simulink model "teste2"  (R2014a)
settings: Solver=ode3  StartTime=0.0  StopTime=80  FixedStep=0.001  RelTol=1e-3
libraries: commchan3 x3, simulink x2
settings Model: Creator=andre  LastModifiedBy=andre

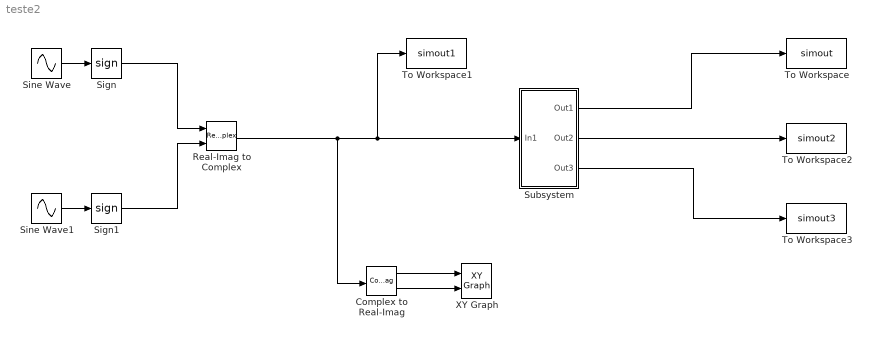
== system teste2 ==
  Complex to Real-Imag : ComplexToRealImag
  Real-Imag to Complex : RealImagToComplex
  Sign : Signum
  Sign1 : Signum
  Sine Wave : Sin  Frequency=10  Phase=0.15  SampleTime=0
  Sine Wave1 : Sin  Frequency=3  Phase=-0.17  SampleTime=0
  Subsystem : Subsystem
  To Workspace : ToWorkspace  VariableName=simout  SampleTime=-1
  To Workspace1 : ToWorkspace  VariableName=simout1  SampleTime=-1
  To Workspace2 : ToWorkspace  VariableName=simout2  SampleTime=-1
  To Workspace3 : ToWorkspace  VariableName=simout3  SampleTime=-1
  XY Graph : simulink/Sinks/XY Graph  xmin=-3  xmax=3  ymin=-3  ymax=3  st=-1
  wires:
  Sine Wave/1 -> Sign/1
  Sine Wave1/1 -> Sign1/1
  Subsystem/1(Out1) -> To Workspace/1
  Subsystem/2(Out2) -> To Workspace2/1
  Subsystem/3(Out3) -> To Workspace3/1
  Sign/1 -> Real-Imag to Complex/1
  Sign1/1 -> Real-Imag to Complex/2
  Complex to Real-Imag/1 -> XY Graph/1
  Complex to Real-Imag/2 -> XY Graph/2
  Real-Imag to Complex/1 -> Complex to Real-Imag/1, To Workspace1/1, Subsystem/1(In1)

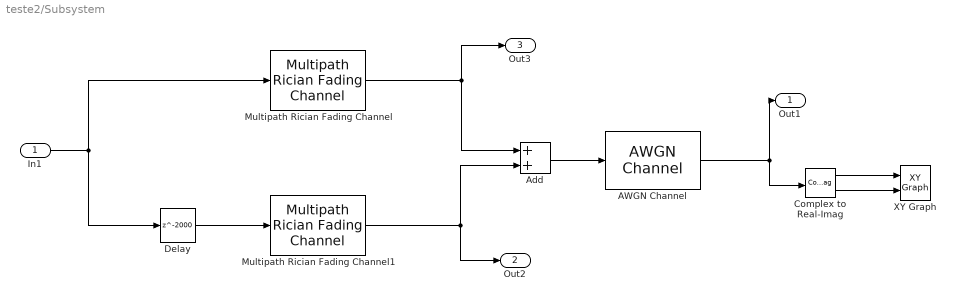
== system teste2/Subsystem ==
  In1 : Inport
  AWGN Channel : commchan3/AWGN Channel  InputProcessing=Inherited (this choice will be removed - see release notes)  seed=67  noiseMode="Signal to noise ratio  (SNR)"  EbNodB=30  EsNodB=10  SNRdB=200  bitsPerSym=1  Ps=1  Tsym=1  variance=1
  Add : Sum
  Complex to Real-Imag : ComplexToRealImag
  Delay : Delay  DelayLength=2000
  Multipath Rician Fading Channel : commchan3/Multipath Rician Fading Channel  K=1  fdLOS=0.001  thetaLOS=0  maxDopplerShift=0.0001  spectrumType=Jakes  sigmaGaussian=1/sqrt(2)  coeffRounded=[1 -1.72 0.785]  freqMinMaxRJakes=[0 1]  freqMinMaxAJakes=[0 1]  sigmaGaussian1=1/sqrt(2)  sigmaGaussian2=1/sqrt(2)  centerFreqGaussian1=0  centerFreqGaussian2=0  gainGaussian1=0.5  gainGaussian2=0.5  coeffBell=9  dopplerSpectrum=doppler.jakes  pathDelays=0  avgPathGaindB=0  normalizePathGains=on  seed=73  enableProbe=0  openVisAtStart=off  outPathGains=off  outDelay=off
  Multipath Rician Fading Channel1 : commchan3/Multipath Rician Fading Channel  K=1  fdLOS=0.01  thetaLOS=0  maxDopplerShift=0.001  spectrumType=Jakes  sigmaGaussian=1/sqrt(2)  coeffRounded=[1 -1.72 0.785]  freqMinMaxRJakes=[0 1]  freqMinMaxAJakes=[0 1]  sigmaGaussian1=1/sqrt(2)  sigmaGaussian2=1/sqrt(2)  centerFreqGaussian1=0  centerFreqGaussian2=0  gainGaussian1=0.5  gainGaussian2=0.5  coeffBell=9  dopplerSpectrum=doppler.jakes  pathDelays=0  avgPathGaindB=0  normalizePathGains=on  seed=31  enableProbe=0  openVisAtStart=off  outPathGains=off  outDelay=off
  XY Graph : simulink/Sinks/XY Graph  xmin=-3  xmax=3  ymin=-3  ymax=3  st=-1
  Out1 : Outport
  Out2 : Outport  Port=2
  Out3 : Outport  Port=3
  wires:
  AWGN Channel/1 -> Out1/1, Complex to Real-Imag/1
  Add/1 -> AWGN Channel/1
  Multipath Rician Fading Channel1/1 -> Add/2, Out2/1
  In1/1 -> Delay/1, Multipath Rician Fading Channel/1
  Multipath Rician Fading Channel/1 -> Add/1, Out3/1
  Delay/1 -> Multipath Rician Fading Channel1/1
  Complex to Real-Imag/1 -> XY Graph/1
  Complex to Real-Imag/2 -> XY Graph/2
